simulink model "c2837x_block_c_function_test"  (R2025b)
settings: Solver=FixedStepDiscrete  StartTime=0.0  StopTime=0.1  FixedStep=0.0001  RelTol=1e-3
settings Model: Creator=Sun  LastModifiedBy=Sun

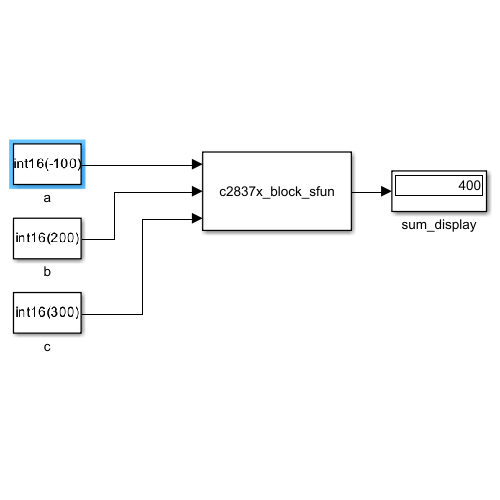
[thumbnail: Simulink's stored preview of the top-level diagram]
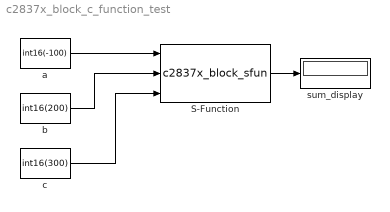
== system c2837x_block_c_function_test ==
  S-Function : S-Function  FunctionName=c2837x_block_sfun  SFunctionDeploymentMode=off  EnableBusSupport=off
  a : Constant  Value=int16(-100)  OutDataTypeStr=int16
  b : Constant  Value=int16(200)  OutDataTypeStr=int16
  c : Constant  Value=int16(300)  OutDataTypeStr=int16
  sum_display : Display
  wires:
  a/1 -> S-Function/1
  b/1 -> S-Function/2
  c/1 -> S-Function/3
  S-Function/1 -> sum_display/1
